simulink model "test_bu01_2018b"  (R2018b)
settings: Solver=FixedStepAuto  StartTime=0.0  StopTime=10  FixedStep=0.02  RelTol=1e-3
model workspace (MAT data in the model file):
  Ixx = 0.8
  Iyy = 2.075
  Izz = 1.25
  K = 0.75
  Mass = 11.5
  b = 0
libraries: simulink x10, aerolibutil x6, vrlib x4, sharedtransform x4, sharedutil x3, shared6dof x1
(part 1 of 4)
settings Model: Creator=Administrator  LastModifiedBy=39926
settings DataIOCC: ReturnWorkspaceOutputs=on

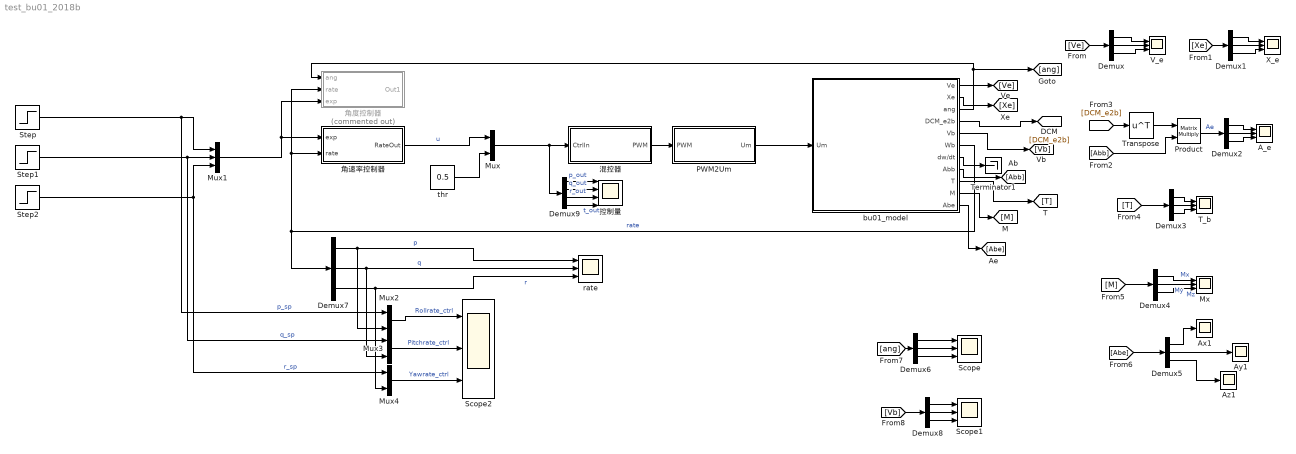
== system test_bu01_2018b ==
  A_e : Scope  NumInputPorts=3
  Ax1 : Scope
  Ay1 : Scope
  Az1 : Scope
  Demux{,1..8} (9 alike) : Demux  Outputs=3
  Demux9 : Demux
  Mux{,2..4} (4 alike) : Mux  Inputs=2
  Mux1 : Mux  Inputs=3
  Mx : Scope  NumInputPorts=3
  PWM2Um : Subsystem
  Product : Product  Multiplication=Matrix(*)
  Scope : Scope  NumInputPorts=3
  Scope1 : Scope  NumInputPorts=3
  Scope2 : Scope  NumInputPorts=3
  Step : Step  SampleTime=0
  Step1 : Step  SampleTime=0
  Step2 : Step  SampleTime=0
  T_b : Scope  NumInputPorts=3
  Terminator1 : Terminator
  Transpose : Math  Operator=transpose  SaturateOnIntegerOverflow=on
  V_e : Scope  NumInputPorts=3
  X_e : Scope  NumInputPorts=3
  bu01_model : Subsystem  mask{Density=1.185}
      mask prompts: Density "空气密度D"
  rate : Scope  NumInputPorts=3
  thr : Constant  Value=0.5
  控制量 : Scope  NumInputPorts=4
  混控器 : Subsystem
  角度控制器 : Subsystem  Commented=on
  角速率控制器 : Subsystem
  wires:
  bu01_model/8(Abb) -> [Abb]
  bu01_model/7(dw/dt) -> Terminator1/1
  bu01_model/4(DCM_e2b) -> [DCM_e2b]
  bu01_model/5(Vb) -> [Vb]
  Mux/1 -> Demux9/1, 混控器/1(CtrlIn)
  bu01_model/3(ang) -> [ang], 角度控制器/1(ang)
  bu01_model/6(Wb) -> Demux7/1, 角速率控制器/2(rate), 角度控制器/2(rate)  "rate"
  Mux1/1 -> 角度控制器/3(exp), 角速率控制器/1(exp)
  thr/1 -> Mux/2
  bu01_model/2(Xe) -> [Xe]
  Demux/1 -> V_e/1
  bu01_model/1(Ve) -> [Ve]
  [Ve] -> Demux/1
  [Xe] -> Demux1/1
  Demux1/1 -> X_e/1
  Demux1/2 -> X_e/2
  Demux1/3 -> X_e/3
  [DCM_e2b] -> Transpose/1
  Transpose/1 -> Product/1
  [Abb] -> Product/2
  Product/1 -> Demux2/1  "Ae"
  Demux2/1 -> A_e/1
  Demux2/2 -> A_e/2
  bu01_model/9(T) -> [T]
  bu01_model/10(M) -> [M]
  Demux3/3 -> T_b/3
  Demux3/2 -> T_b/2
  Demux3/1 -> T_b/1
  [T] -> Demux3/1
  [M] -> Demux4/1
  Demux4/1 -> Mx/1  "Mx"
  Demux4/2 -> Mx/2  "My"
  Demux4/3 -> Mx/3  "Mz"
  Demux2/3 -> A_e/3
  bu01_model/11(Abe) -> [Abe]
  Demux5/3 -> Az1/1
  Demux5/2 -> Ay1/1
  Demux5/1 -> Ax1/1
  [Abe] -> Demux5/1
  Step/1 -> Mux2/1, Mux1/1  "p_sp"
  Step1/1 -> Mux3/1, Mux1/2  "q_sp"
  Step2/1 -> Mux4/1, Mux1/3  "r_sp"
  Demux/2 -> V_e/2
  Demux/3 -> V_e/3
  [ang] -> Demux6/1
  Demux6/1 -> Scope/1
  Demux6/2 -> Scope/2
  Demux6/3 -> Scope/3
  PWM2Um/1(Um) -> bu01_model/1(Um)
  混控器/1(PWM) -> PWM2Um/1(PWM)
  Demux7/1 -> Mux2/2, rate/1  "p"
  Demux7/2 -> Mux3/2, rate/2  "q"
  Demux7/3 -> Mux4/2, rate/3  "r"
  [Vb] -> Demux8/1
  Demux8/1 -> Scope1/1
  Demux8/2 -> Scope1/2
  Demux8/3 -> Scope1/3
  Mux2/1 -> Scope2/1  "Rollrate_ctrl"
  Mux3/1 -> Scope2/2  "Pitchrate_ctrl"
  Mux4/1 -> Scope2/3  "Yawrate_ctrl"
  Demux9/1 -> 控制量/1  "p_out"
  Demux9/2 -> 控制量/2  "q_out"
  Demux9/3 -> 控制量/3  "r_out"
  Demux9/4 -> 控制量/4  "t_out"
  角速率控制器/1(RateOut) -> Mux/1  "u"

== system test_bu01_2018b/PWM2Um ==
  PWM : Inport
  Add : Sum  Inputs=+-
  Add1 : Sum  Inputs=+-
  Constant : Constant  Value=36.092
  Constant1 : Constant  Value=36.491
  Demux : Demux  Outputs=2
  Demux1 : Demux  Outputs=8
  Gain : Gain  Gain=0.0333
  Gain1 : Gain  Gain=0.0355
  Mux : Mux  Inputs=2
  Saturation : Saturate  UpperLimit=1900  LowerLimit=1200
  Scope : Scope  NumInputPorts=8
  Um : Outport
  wires:
  Demux/1 -> Gain/1
  Gain/1 -> Add/1
  Constant/1 -> Add/2
  Demux/2 -> Gain1/1
  Saturation/1 -> Demux/1
  PWM/1 -> Saturation/1
  Gain1/1 -> Add1/1
  Constant1/1 -> Add1/2
  Add1/1 -> Mux/2
  Add/1 -> Mux/1
  Mux/1 -> Demux1/1, Um/1
  Demux1/1 -> Scope/1
  Demux1/2 -> Scope/2
  Demux1/3 -> Scope/3
  Demux1/4 -> Scope/4
  Demux1/5 -> Scope/5
  Demux1/6 -> Scope/6
  Demux1/7 -> Scope/7
  Demux1/8 -> Scope/8

== system test_bu01_2018b/bu01_model ==
  Um : Inport
  6DOF (Quaternion) : shared6dof/6DOF (Euler Angles)  units=Metric (MKS)  mtype=Fixed  rep=Quaternion  xme_0=[0 0 0]  Vm_0=[0 0 0]  eul_0=[0 0 0]  pm_0=[0 0 0]  mass_0=Mass  mass_e=0.5  mass_f=2.0  inertia=[Ixx 0 0; 0 Iyy 0;0 0 Izz]  inertia_e=eye(3)  inertia_f=2*eye(3)  k_quat=1.0  vre_flag=on  abi_flag=on  aMode=0  xme_statename=''  Vm_statename=''  eul_statename=''  quat_statename=''  pm_statename=''  mass_statename=''
      settings: SourceProductBaseCode=AE
  Add : Sum  Inputs=3
  Add1 : Sum
  Constant : Constant  Value=Density
  Constant1 : Constant  Value=[0 0 0]
  Constant2 : Constant  Value=[0 0 0]
  动力系统模型 : Subsystem
  空气动力模型 : ModelReference  ModelNameDialog=BU01AM.slx  SimulationMode=Normal  ModelReferenceVersion=1.55
  重力模型 : Subsystem  mask{G=9.81, m=11.5}
      mask prompts: G "重力加速度G"; m "质量m"
  Ve : Outport
  Xe : Outport  Port=2
  ang : Outport  Port=3
  DCM_e2b : Outport  Port=4
  Vb : Outport  Port=5
  Wb : Outport  Port=6
  dw/dt : Outport  Port=7
  Abb : Outport  Port=8
  T : Outport  Port=9
  M : Outport  Port=10
  Abe : Outport  Port=11
  wires:
  Add1/1 -> M/1, 6DOF (Quaternion)/2  "M"
  6DOF (Quaternion)/1 -> Ve/1
  6DOF (Quaternion)/3 -> ang/1
  6DOF (Quaternion)/2 -> Xe/1
  6DOF (Quaternion)/4 -> 重力模型/1(DCM_e2b), DCM_e2b/1
  Add/1 -> T/1, 6DOF (Quaternion)/1  "T"
  6DOF (Quaternion)/7 -> dw/dt/1
  6DOF (Quaternion)/8 -> Abb/1
  6DOF (Quaternion)/5 -> Vb/1
  6DOF (Quaternion)/6 -> Wb/1, 空气动力模型/2
  Um/1 -> 动力系统模型/1("Um ")
  6DOF (Quaternion)/9 -> Abe/1
  Constant/1 -> 空气动力模型/4
  重力模型/1(Fb_mg) -> Add/1
  动力系统模型/1(Fb) -> Add/2
  空气动力模型/1 -> Add/3
  空气动力模型/2 -> Add1/2
  动力系统模型/2(Mb) -> Add1/1
  Constant1/1 -> 空气动力模型/3, 动力系统模型/3(Wb)
  Constant2/1 -> 空气动力模型/1, 动力系统模型/2(Vb)

== system test_bu01_2018b/混控器 ==
  note: 机体构型描述：
      |           ^
      |           ||
      | 1P   -  ||  -   4N
      | 2N   -  ||  -   3P
      |            ||
      |            ||
      | -------------------
      | 5N  6N   7N 8N
  CtrlIn : Inport
  Add : Sum
  Bias{1..4} (4 alike) : Bias  Bias=[0 b 0 b]
  Constant : Constant  Value=1200
  Demux : Demux  Outputs=8
  Gain : Gain  Gain="[1 1  -1 1]"
  Gain1 : Gain  Gain="[1 0  1 1]"
  Gain{7,9..11} (4 alike) : Gain  Gain=K
  Gain12 : Gain  Gain=700
  Gain2 : Gain  Gain=[-1 0 -1 1]
  Gain3 : Gain  Gain=[-1 1 1 1]
  Gain{4..6,8} (4 alike) : Gain  Gain=[0 -1 0 1]
  Mux : Mux  Inputs=8
  Saturation : Saturate  UpperLimit=1  LowerLimit=0
  Scope : Scope
  Scope1 : Scope  NumInputPorts=8
  Sum of Elements{,1..7} (8 alike) : Sum  Inputs=+
  PWM : Outport
  wires:
  Sum of Elements/1 -> Mux/1
  Gain/1 -> Sum of Elements/1
  Gain2/1 -> Sum of Elements2/1
  Gain3/1 -> Sum of Elements3/1
  Gain1/1 -> Sum of Elements1/1
  Bias3/1 -> Sum of Elements7/1
  Saturation/1 -> Gain12/1, Demux/1
  Sum of Elements1/1 -> Mux/2
  Sum of Elements2/1 -> Mux/3
  Sum of Elements3/1 -> Mux/4
  Sum of Elements4/1 -> Mux/5
  Sum of Elements5/1 -> Mux/6
  Sum of Elements6/1 -> Mux/7
  Sum of Elements7/1 -> Mux/8
  CtrlIn/1 -> Scope/1, Gain3/1, Gain4/1, Gain5/1, Gain8/1, Gain6/1, Gain1/1, Gain/1, Gain2/1
  Demux/1 -> Scope1/1  "m1"
  Demux/2 -> Scope1/2  "m2"
  Demux/3 -> Scope1/3  "m3"
  Demux/4 -> Scope1/4  "m4"
  Demux/5 -> Scope1/5  "m5"
  Demux/6 -> Scope1/6  "m6"
  Demux/7 -> Scope1/7  "m7"
  Demux/8 -> Scope1/8  "m8"
  Gain7/1 -> Bias3/1
  Gain8/1 -> Gain7/1
  Bias1/1 -> Sum of Elements6/1
  Gain6/1 -> Gain9/1
  Gain9/1 -> Bias1/1
  Bias2/1 -> Sum of Elements5/1
  Gain5/1 -> Gain10/1
  Gain10/1 -> Bias2/1
  Bias4/1 -> Sum of Elements4/1
  Gain4/1 -> Gain11/1
  Gain11/1 -> Bias4/1
  Gain12/1 -> Add/1
  Constant/1 -> Add/2
  Add/1 -> PWM/1
  Mux/1 -> Saturation/1

== system test_bu01_2018b/角度控制器 ==
  ang : Inport
  rate : Inport  Port=2
  exp : Inport  Port=3
  Demux : Demux  Outputs=3
  Demux1 : Demux  Outputs=3
  Demux2 : Demux  Outputs=3
  Mux : Mux  Inputs=3
  Mux1 : Mux  Inputs=2
  Mux2 : Mux  Inputs=2
  Mux3 : Mux  Inputs=2
  Mux4 : Mux  Inputs=3
  PID Controller : simulink/Continuous/PID Controller  Controller=PID  Form=Parallel  TimeDomain=Continuous-time  SampleTime=-1  IntegratorMethod=Forward Euler  FilterMethod=Forward Euler  ControllerParametersSource=internal  P=0.1  I=0.1  D=0  UseFilter=on  N=100  TunerSelectOption=Transfer Function Based (PID Tuner App)  InitialConditionSource=internal  InitialConditionForIntegrator=0  InitialConditionForFilter=0  DifferentiatorICPrevScaledInput=0  ExternalReset=none  TrackingMode=off  Kt=1  LimitOutput=off  UpperSaturationLimit=inf  LowerSaturationLimit=-inf  LinearizeAsGain=on  AntiWindupMode=none  Kb=1  POutMin=[]  POutMax=[]  IOutMin=[]  IOutMax=[]  DOutMin=[]  DOutMax=[]  NOutMin=[]  NOutMax=[]  SumOutMin=[]  SumOutMax=[]  SaturationOutMin=[]  SaturationOutMax=[]  PParamMin=[]  PParamMax=[]  IParamMin=[]  IParamMax=[]  DParamMin=[]  DParamMax=[]  NParamMin=[]  NParamMax=[]  KbParamMin=[]  KbParamMax=[]  KtParamMin=[]  KtParamMax=[]  KbOutMin=[]  KbOutMax=[]  KtOutMin=[]  KtOutMax=[]  IntegratorOutMin=[]  IntegratorOutMax=[]  FilterOutMin=[]  FilterOutMax=[]  SumI1OutMin=[]  SumI1OutMax=[]  SumI2OutMin=[]  SumI2OutMax=[]  SumI3OutMin=[]  SumI3OutMax=[]  SumI4OutMin=[]  SumI4OutMax=[]  SumDOutMin=[]  SumDOutMax=[]  DifferentiatorOutMin=[]  DifferentiatorOutMax=[]  FilterDiffOutCoefMin=[]  FilterDiffOutCoefMax=[]  ReciprocalOutMin=[]  ReciprocalOutMax=[]  SumDenOutMin=[]  SumDenOutMax=[]  SumNumOutMin=[]  SumNumOutMax=[]  DivideOutMin=[]  DivideOutMax=[]  IntegratorContinuousStateAttributes=''  IntegratorStateMustResolveToSignalObject=off  IntegratorRTWStateStorageClass=Auto  FilterContinuousStateAttributes=''  FilterStateMustResolveToSignalObject=off  FilterRTWStateStorageClass=Auto  ParallelPVariant=InternalParameters  IdealPVariant=Disabled  IVariant=InternalParameters  DVariant=InternalParameters  IntegratorVariant=Continuous  SatVariant=Disabled  AWVariant=Passthrough  PCopyVariant=Disabled  TRVariant=Disabled  FdbkBlocksVariant=Forward  IdealPFdbkVariant=Disabled  SatFdbkVariant=Disabled  DerivativeFilterVariant=ContFilter  NVariant=InternalParameters  NCopyVariant=Disabled  FilterICVariant=InternalICsFilter  IntegratorICVariant=InternalICs  ExternalResetVariant=Disabled  TRSumVariant=Passthrough  SumFdbkVariant=Disabled  SumVariant=Sum_PID
  PID Controller1 : simulink/Continuous/PID Controller  Controller=PID  Form=Parallel  TimeDomain=Continuous-time  SampleTime=-1  IntegratorMethod=Forward Euler  FilterMethod=Forward Euler  ControllerParametersSource=internal  P=0.15  I=0.1  D=0  UseFilter=on  N=100  TunerSelectOption=Transfer Function Based (PID Tuner App)  InitialConditionSource=internal  InitialConditionForIntegrator=0  InitialConditionForFilter=0  DifferentiatorICPrevScaledInput=0  ExternalReset=none  TrackingMode=off  Kt=1  LimitOutput=off  UpperSaturationLimit=inf  LowerSaturationLimit=-inf  LinearizeAsGain=on  AntiWindupMode=none  Kb=1  POutMin=[]  POutMax=[]  IOutMin=[]  IOutMax=[]  DOutMin=[]  DOutMax=[]  NOutMin=[]  NOutMax=[]  SumOutMin=[]  SumOutMax=[]  SaturationOutMin=[]  SaturationOutMax=[]  PParamMin=[]  PParamMax=[]  IParamMin=[]  IParamMax=[]  DParamMin=[]  DParamMax=[]  NParamMin=[]  NParamMax=[]  KbParamMin=[]  KbParamMax=[]  KtParamMin=[]  KtParamMax=[]  KbOutMin=[]  KbOutMax=[]  KtOutMin=[]  KtOutMax=[]  IntegratorOutMin=[]  IntegratorOutMax=[]  FilterOutMin=[]  FilterOutMax=[]  SumI1OutMin=[]  SumI1OutMax=[]  SumI2OutMin=[]  SumI2OutMax=[]  SumI3OutMin=[]  SumI3OutMax=[]  SumI4OutMin=[]  SumI4OutMax=[]  SumDOutMin=[]  SumDOutMax=[]  DifferentiatorOutMin=[]  DifferentiatorOutMax=[]  FilterDiffOutCoefMin=[]  FilterDiffOutCoefMax=[]  ReciprocalOutMin=[]  ReciprocalOutMax=[]  SumDenOutMin=[]  SumDenOutMax=[]  SumNumOutMin=[]  SumNumOutMax=[]  DivideOutMin=[]  DivideOutMax=[]  IntegratorContinuousStateAttributes=''  IntegratorStateMustResolveToSignalObject=off  IntegratorRTWStateStorageClass=Auto  FilterContinuousStateAttributes=''  FilterStateMustResolveToSignalObject=off  FilterRTWStateStorageClass=Auto  ParallelPVariant=InternalParameters  IdealPVariant=Disabled  IVariant=InternalParameters  DVariant=InternalParameters  IntegratorVariant=Continuous  SatVariant=Disabled  AWVariant=Passthrough  PCopyVariant=Disabled  TRVariant=Disabled  FdbkBlocksVariant=Forward  IdealPFdbkVariant=Disabled  SatFdbkVariant=Disabled  DerivativeFilterVariant=ContFilter  NVariant=InternalParameters  NCopyVariant=Disabled  FilterICVariant=InternalICsFilter  IntegratorICVariant=InternalICs  ExternalResetVariant=Disabled  TRSumVariant=Passthrough  SumFdbkVariant=Disabled  SumVariant=Sum_PID
  PID Controller2 : simulink/Continuous/PID Controller  Controller=PID  Form=Parallel  TimeDomain=Continuous-time  SampleTime=-1  IntegratorMethod=Forward Euler  FilterMethod=Forward Euler  ControllerParametersSource=internal  P=0.3  I=0.1  D=0  UseFilter=on  N=100  TunerSelectOption=Transfer Function Based (PID Tuner App)  InitialConditionSource=internal  InitialConditionForIntegrator=0  InitialConditionForFilter=0  DifferentiatorICPrevScaledInput=0  ExternalReset=none  TrackingMode=off  Kt=1  LimitOutput=off  UpperSaturationLimit=inf  LowerSaturationLimit=-inf  LinearizeAsGain=on  AntiWindupMode=none  Kb=1  POutMin=[]  POutMax=[]  IOutMin=[]  IOutMax=[]  DOutMin=[]  DOutMax=[]  NOutMin=[]  NOutMax=[]  SumOutMin=[]  SumOutMax=[]  SaturationOutMin=[]  SaturationOutMax=[]  PParamMin=[]  PParamMax=[]  IParamMin=[]  IParamMax=[]  DParamMin=[]  DParamMax=[]  NParamMin=[]  NParamMax=[]  KbParamMin=[]  KbParamMax=[]  KtParamMin=[]  KtParamMax=[]  KbOutMin=[]  KbOutMax=[]  KtOutMin=[]  KtOutMax=[]  IntegratorOutMin=[]  IntegratorOutMax=[]  FilterOutMin=[]  FilterOutMax=[]  SumI1OutMin=[]  SumI1OutMax=[]  SumI2OutMin=[]  SumI2OutMax=[]  SumI3OutMin=[]  SumI3OutMax=[]  SumI4OutMin=[]  SumI4OutMax=[]  SumDOutMin=[]  SumDOutMax=[]  DifferentiatorOutMin=[]  DifferentiatorOutMax=[]  FilterDiffOutCoefMin=[]  FilterDiffOutCoefMax=[]  ReciprocalOutMin=[]  ReciprocalOutMax=[]  SumDenOutMin=[]  SumDenOutMax=[]  SumNumOutMin=[]  SumNumOutMax=[]  DivideOutMin=[]  DivideOutMax=[]  IntegratorContinuousStateAttributes=''  IntegratorStateMustResolveToSignalObject=off  IntegratorRTWStateStorageClass=Auto  FilterContinuousStateAttributes=''  FilterStateMustResolveToSignalObject=off  FilterRTWStateStorageClass=Auto  ParallelPVariant=InternalParameters  IdealPVariant=Disabled  IVariant=InternalParameters  DVariant=InternalParameters  IntegratorVariant=Continuous  SatVariant=Disabled  AWVariant=Passthrough  PCopyVariant=Disabled  TRVariant=Disabled  FdbkBlocksVariant=Forward  IdealPFdbkVariant=Disabled  SatFdbkVariant=Disabled  DerivativeFilterVariant=ContFilter  NVariant=InternalParameters  NCopyVariant=Disabled  FilterICVariant=InternalICsFilter  IntegratorICVariant=InternalICs  ExternalResetVariant=Disabled  TRSumVariant=Passthrough  SumFdbkVariant=Disabled  SumVariant=Sum_PID
  Product : Product
  Saturation : Saturate  UpperLimit=1  LowerLimit=-1
  Scope : Scope  NumInputPorts=3
  Scope1 : Scope
  Scope2 : Scope
  Subsystem : Subsystem
  Sum : Sum  Inputs=|+-
  pitch gain : Constant
  roll gain : Constant
  yaw gain : Constant
  求取航向衰减后的期望四元数 : Subsystem
  求取角度误差 : Subsystem
  Out1 : Outport
  wires:
  ang/1 -> Demux/1, 求取航向衰减后的期望四元数/1(ang)
  exp/1 -> Demux1/1, 求取航向衰减后的期望四元数/2(exp)
  roll gain/1 -> Mux/1, Subsystem/1(roll_gain)
  pitch gain/1 -> Subsystem/2("pitch_gain "), Mux/2
  yaw gain/1 -> Subsystem/3(yaw_gain), Mux/3
  Subsystem/1(yaw_w) -> 求取航向衰减后的期望四元数/3("yaw_w ")
  求取航向衰减后的期望四元数/1(q) -> 求取角度误差/1(q)
  求取航向衰减后的期望四元数/2(qd) -> 求取角度误差/2(qd)
  求取角度误差/1(rpy_err) -> Product/1
  Mux/1 -> Product/2
  Product/1 -> Sum/1  "rate_sp"
  rate/1 -> Sum/2
  Sum/1 -> Scope1/1, Demux2/1
  Mux4/1 -> Scope2/1, Saturation/1
  Saturation/1 -> Out1/1
  Demux/1 -> Mux1/1  "roll"
  Demux1/1 -> Mux1/2  "roll_sp"
  Demux/2 -> Mux2/1  "pitch"
  Demux1/2 -> Mux2/2  "pitch_sp"
  Demux/3 -> Mux3/1  "yaw"
  Demux1/3 -> Mux3/2  "yaw_sp"
  Mux1/1 -> Scope/1
  Mux2/1 -> Scope/2
  Mux3/1 -> Scope/3
  Demux2/1 -> PID Controller/1
  Demux2/2 -> PID Controller1/1
  Demux2/3 -> PID Controller2/1
  PID Controller/1 -> Mux4/1
  PID Controller1/1 -> Mux4/2
  PID Controller2/1 -> Mux4/3

== system test_bu01_2018b/角速率控制器 ==
  exp : Inport
  rate : Inport  Port=2
  " roll-off" : TransferFcn  Numerator=[40]  Denominator=[1 40]
  " roll-off1" : TransferFcn  Numerator=[40]  Denominator=[1 40]
  " roll-off2" : TransferFcn  Numerator=[40]  Denominator=[1 40]
  Demux : Demux  Outputs=3
  Mux : Mux  Inputs=3
  PID Controller : simulink/Continuous/PID Controller  Controller=PI  Form=Parallel  TimeDomain=Continuous-time  SampleTime=-1  IntegratorMethod=Forward Euler  FilterMethod=Forward Euler  ControllerParametersSource=internal  P=0.1  I=0.01  D=0.001  UseFilter=on  N=100  TunerSelectOption=Transfer Function Based (PID Tuner App)  InitialConditionSource=internal  InitialConditionForIntegrator=0  InitialConditionForFilter=0  DifferentiatorICPrevScaledInput=0  ExternalReset=none  TrackingMode=off  Kt=1  LimitOutput=off  UpperSaturationLimit=1  LowerSaturationLimit=-1  LinearizeAsGain=on  AntiWindupMode=none  Kb=1  POutMin=[]  POutMax=[]  IOutMin=[]  IOutMax=[]  DOutMin=[]  DOutMax=[]  NOutMin=[]  NOutMax=[]  SumOutMin=[]  SumOutMax=[]  SaturationOutMin=[]  SaturationOutMax=[]  PParamMin=[]  PParamMax=[]  IParamMin=[]  IParamMax=[]  DParamMin=[]  DParamMax=[]  NParamMin=[]  NParamMax=[]  KbParamMin=[]  KbParamMax=[]  KtParamMin=[]  KtParamMax=[]  KbOutMin=[]  KbOutMax=[]  KtOutMin=[]  KtOutMax=[]  IntegratorOutMin=[]  IntegratorOutMax=[]  FilterOutMin=[]  FilterOutMax=[]  SumI1OutMin=[]  SumI1OutMax=[]  SumI2OutMin=[]  SumI2OutMax=[]  SumI3OutMin=[]  SumI3OutMax=[]  SumI4OutMin=[]  SumI4OutMax=[]  SumDOutMin=[]  SumDOutMax=[]  DifferentiatorOutMin=[]  DifferentiatorOutMax=[]  FilterDiffOutCoefMin=[]  FilterDiffOutCoefMax=[]  ReciprocalOutMin=[]  ReciprocalOutMax=[]  SumDenOutMin=[]  SumDenOutMax=[]  SumNumOutMin=[]  SumNumOutMax=[]  DivideOutMin=[]  DivideOutMax=[]  IntegratorContinuousStateAttributes=''  IntegratorStateMustResolveToSignalObject=off  IntegratorRTWStateStorageClass=Auto  FilterContinuousStateAttributes=''  FilterStateMustResolveToSignalObject=off  FilterRTWStateStorageClass=Auto  ParallelPVariant=InternalParameters  IdealPVariant=Disabled  IVariant=InternalParameters  DVariant=Disabled  IntegratorVariant=Continuous  SatVariant=Disabled  AWVariant=Passthrough  PCopyVariant=Disabled  TRVariant=Disabled  FdbkBlocksVariant=Forward  IdealPFdbkVariant=Disabled  SatFdbkVariant=Disabled  DerivativeFilterVariant=Disabled  NVariant=Disabled  NCopyVariant=Disabled_SignalSpec  FilterICVariant=Disabled  IntegratorICVariant=InternalICs  ExternalResetVariant=Disabled  TRSumVariant=Passthrough  SumFdbkVariant=Disabled  SumVariant=Sum_PI
  PID Controller1 : simulink/Continuous/PID Controller  Controller=PI  Form=Parallel  TimeDomain=Continuous-time  SampleTime=-1  IntegratorMethod=Forward Euler  FilterMethod=Forward Euler  ControllerParametersSource=internal  P=0.1  I=0.01  D=0  UseFilter=on  N=100  TunerSelectOption=Transfer Function Based (PID Tuner App)  InitialConditionSource=internal  InitialConditionForIntegrator=0  InitialConditionForFilter=0  DifferentiatorICPrevScaledInput=0  ExternalReset=none  TrackingMode=off  Kt=1  LimitOutput=off  UpperSaturationLimit=1  LowerSaturationLimit=-1  LinearizeAsGain=on  AntiWindupMode=none  Kb=1  POutMin=[]  POutMax=[]  IOutMin=[]  IOutMax=[]  DOutMin=[]  DOutMax=[]  NOutMin=[]  NOutMax=[]  SumOutMin=[]  SumOutMax=[]  SaturationOutMin=[]  SaturationOutMax=[]  PParamMin=[]  PParamMax=[]  IParamMin=[]  IParamMax=[]  DParamMin=[]  DParamMax=[]  NParamMin=[]  NParamMax=[]  KbParamMin=[]  KbParamMax=[]  KtParamMin=[]  KtParamMax=[]  KbOutMin=[]  KbOutMax=[]  KtOutMin=[]  KtOutMax=[]  IntegratorOutMin=[]  IntegratorOutMax=[]  FilterOutMin=[]  FilterOutMax=[]  SumI1OutMin=[]  SumI1OutMax=[]  SumI2OutMin=[]  SumI2OutMax=[]  SumI3OutMin=[]  SumI3OutMax=[]  SumI4OutMin=[]  SumI4OutMax=[]  SumDOutMin=[]  SumDOutMax=[]  DifferentiatorOutMin=[]  DifferentiatorOutMax=[]  FilterDiffOutCoefMin=[]  FilterDiffOutCoefMax=[]  ReciprocalOutMin=[]  ReciprocalOutMax=[]  SumDenOutMin=[]  SumDenOutMax=[]  SumNumOutMin=[]  SumNumOutMax=[]  DivideOutMin=[]  DivideOutMax=[]  IntegratorContinuousStateAttributes=''  IntegratorStateMustResolveToSignalObject=off  IntegratorRTWStateStorageClass=Auto  FilterContinuousStateAttributes=''  FilterStateMustResolveToSignalObject=off  FilterRTWStateStorageClass=Auto  ParallelPVariant=InternalParameters  IdealPVariant=Disabled  IVariant=InternalParameters  DVariant=Disabled  IntegratorVariant=Continuous  SatVariant=Disabled  AWVariant=Passthrough  PCopyVariant=Disabled  TRVariant=Disabled  FdbkBlocksVariant=Forward  IdealPFdbkVariant=Disabled  SatFdbkVariant=Disabled  DerivativeFilterVariant=Disabled  NVariant=Disabled  NCopyVariant=Disabled_SignalSpec  FilterICVariant=Disabled  IntegratorICVariant=InternalICs  ExternalResetVariant=Disabled  TRSumVariant=Passthrough  SumFdbkVariant=Disabled  SumVariant=Sum_PI
  PID Controller2 : simulink/Continuous/PID Controller  Controller=PI  Form=Parallel  TimeDomain=Continuous-time  SampleTime=-1  IntegratorMethod=Forward Euler  FilterMethod=Forward Euler  ControllerParametersSource=internal  P=0.1  I=0.01  D=0  UseFilter=on  N=100  TunerSelectOption=Transfer Function Based (PID Tuner App)  InitialConditionSource=internal  InitialConditionForIntegrator=0  InitialConditionForFilter=0  DifferentiatorICPrevScaledInput=0  ExternalReset=none  TrackingMode=off  Kt=1  LimitOutput=off  UpperSaturationLimit=1  LowerSaturationLimit=-1  LinearizeAsGain=on  AntiWindupMode=none  Kb=1  POutMin=[]  POutMax=[]  IOutMin=[]  IOutMax=[]  DOutMin=[]  DOutMax=[]  NOutMin=[]  NOutMax=[]  SumOutMin=[]  SumOutMax=[]  SaturationOutMin=[]  SaturationOutMax=[]  PParamMin=[]  PParamMax=[]  IParamMin=[]  IParamMax=[]  DParamMin=[]  DParamMax=[]  NParamMin=[]  NParamMax=[]  KbParamMin=[]  KbParamMax=[]  KtParamMin=[]  KtParamMax=[]  KbOutMin=[]  KbOutMax=[]  KtOutMin=[]  KtOutMax=[]  IntegratorOutMin=[]  IntegratorOutMax=[]  FilterOutMin=[]  FilterOutMax=[]  SumI1OutMin=[]  SumI1OutMax=[]  SumI2OutMin=[]  SumI2OutMax=[]  SumI3OutMin=[]  SumI3OutMax=[]  SumI4OutMin=[]  SumI4OutMax=[]  SumDOutMin=[]  SumDOutMax=[]  DifferentiatorOutMin=[]  DifferentiatorOutMax=[]  FilterDiffOutCoefMin=[]  FilterDiffOutCoefMax=[]  ReciprocalOutMin=[]  ReciprocalOutMax=[]  SumDenOutMin=[]  SumDenOutMax=[]  SumNumOutMin=[]  SumNumOutMax=[]  DivideOutMin=[]  DivideOutMax=[]  IntegratorContinuousStateAttributes=''  IntegratorStateMustResolveToSignalObject=off  IntegratorRTWStateStorageClass=Auto  FilterContinuousStateAttributes=''  FilterStateMustResolveToSignalObject=off  FilterRTWStateStorageClass=Auto  ParallelPVariant=InternalParameters  IdealPVariant=Disabled  IVariant=InternalParameters  DVariant=Disabled  IntegratorVariant=Continuous  SatVariant=Disabled  AWVariant=Passthrough  PCopyVariant=Disabled  TRVariant=Disabled  FdbkBlocksVariant=Forward  IdealPFdbkVariant=Disabled  SatFdbkVariant=Disabled  DerivativeFilterVariant=Disabled  NVariant=Disabled  NCopyVariant=Disabled_SignalSpec  FilterICVariant=Disabled  IntegratorICVariant=InternalICs  ExternalResetVariant=Disabled  TRSumVariant=Passthrough  SumFdbkVariant=Disabled  SumVariant=Sum_PI
  Sum : Sum  Inputs=|+-
  RateOut : Outport
  wires:
  Mux/1 -> RateOut/1
  exp/1 -> Sum/1
  rate/1 -> Sum/2
  Sum/1 -> Demux/1
  Demux/1 -> PID Controller/1
  Demux/2 -> PID Controller1/1
  Demux/3 -> PID Controller2/1
  PID Controller/1 -> " roll-off"/1
  " roll-off"/1 -> Mux/1
  " roll-off1"/1 -> Mux/2
  PID Controller1/1 -> " roll-off1"/1
  PID Controller2/1 -> " roll-off2"/1
  " roll-off2"/1 -> Mux/3

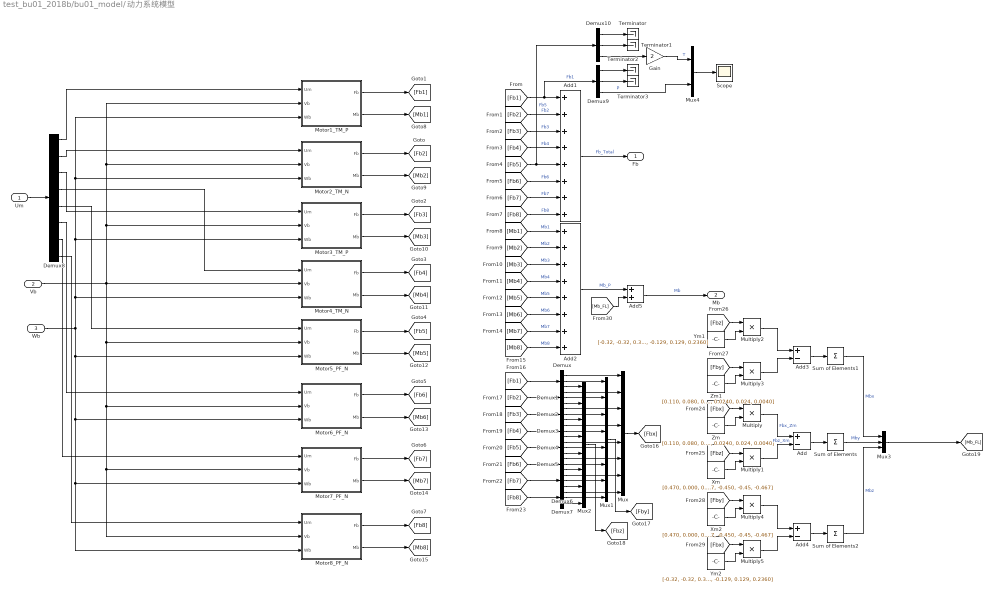
== system test_bu01_2018b/bu01_model/动力系统模型 ==
  "Um " : Inport
  Vb : Inport  Port=2
  Wb : Inport  Port=3
  Add : Sum  Inputs=+-
  Add1 : Sum  Inputs=8
  Add2 : Sum  Inputs=8
  Add3 : Sum  Inputs=+-
  Add4 : Sum  Inputs=+-
  Add5 : Sum
  Demux{,1..7,9..10} (10 alike) : Demux  Outputs=3
  Demux8 : Demux  Outputs=8
  Gain : Gain  Gain=2
  Motor1_TM_P : Subsystem
  Motor2_TM_N : Subsystem
  Motor3_TM_P : Subsystem
  Motor4_TM_N : Subsystem
  Motor5_PF_N : Subsystem
  Motor6_PF_N : Subsystem
  Motor7_PF_N : Subsystem
  Motor8_PF_N : Subsystem
  Multiply{,1..5} (6 alike) : Product
  Mux : Mux  Inputs=8
  Mux1 : Mux  Inputs=8
  Mux2 : Mux  Inputs=8
  Mux3 : Mux  Inputs=3
  Mux4 : Mux  Inputs=2
  Scope : Scope
  Sum of Elements : Sum  Inputs=+
  Sum of Elements1 : Sum  Inputs=+
  Sum of Elements2 : Sum  Inputs=+
  Terminator{,1..3} (4 alike) : Terminator
  Xm : Constant  Value=[0.470, 0.000, 0.00, 0.47, -0.467, -0.450, -0.45, -0.467]
  Xm2 : Constant  Value=[0.470, 0.000, 0.00, 0.47, -0.467, -0.450, -0.45, -0.467]
  Ym1 : Constant  Value=[-0.32, -0.32, 0.32, 0.32, -0.236, -0.129, 0.129, 0.2360]
  Ym2 : Constant  Value=[-0.32, -0.32, 0.32, 0.32, -0.236, -0.129, 0.129, 0.2360]
  Zm : Constant  Value=[0.110, 0.080, 0.08, 0.11, 0.0040, 0.0240, 0.024, 0.0040]
  Zm1 : Constant  Value=[0.110, 0.080, 0.08, 0.11, 0.0040, 0.0240, 0.024, 0.0040]
  Fb : Outport
  Mb : Outport  Port=2
  wires:
  Mux4/1 -> Scope/1
  Gain/1 -> Mux4/1  "T"
  Demux10/3 -> Gain/1
  Demux9/3 -> Mux4/2  "P"
  Demux9/2 -> Terminator3/1
  Demux9/1 -> Terminator2/1
  Demux10/2 -> Terminator1/1
  Demux10/1 -> Terminator/1
  Vb/1 -> Motor4_TM_N/2(Vb), Motor3_TM_P/2(Vb), Motor1_TM_P/2(Vb), Motor2_TM_N/2(Vb), Motor5_PF_N/2(Vb), Motor6_PF_N/2(Vb), Motor8_PF_N/2(Vb), Motor7_PF_N/2(Vb)
  Wb/1 -> Motor5_PF_N/3(Wb), Motor6_PF_N/3(Wb), Motor8_PF_N/3(Wb), Motor7_PF_N/3(Wb), Motor4_TM_N/3(Wb), Motor3_TM_P/3(Wb), Motor1_TM_P/3(Wb), Motor2_TM_N/3(Wb)
  Motor1_TM_P/1(Fb) -> [Fb1]
  Motor2_TM_N/1(Fb) -> [Fb2]
  Motor3_TM_P/1(Fb) -> [Fb3]
  Motor4_TM_N/1(Fb) -> [Fb4]
  Motor5_PF_N/1(Fb) -> [Fb5]
  Motor6_PF_N/1(Fb) -> [Fb6]
  Motor7_PF_N/1(Fb) -> [Fb7]
  Motor8_PF_N/1(Fb) -> [Fb8]
  Motor1_TM_P/2(Mb) -> [Mb1]
  Motor3_TM_P/2(Mb) -> [Mb3]
  Motor4_TM_N/2(Mb) -> [Mb4]
  Motor5_PF_N/2(Mb) -> [Mb5]
  Motor6_PF_N/2(Mb) -> [Mb6]
  Motor7_PF_N/2(Mb) -> [Mb7]
  Motor8_PF_N/2(Mb) -> [Mb8]
  [Fb8] -> Add1/8  "Fb8"
  [Fb7] -> Add1/7  "Fb7"
  [Fb6] -> Add1/6  "Fb6"
  [Fb5] -> Add1/5, Demux10/1  "Fb5"
  [Fb4] -> Add1/4  "Fb4"
  [Fb3] -> Add1/3  "Fb3"
  [Fb2] -> Add1/2  "Fb2"
  [Fb1] -> Add1/1, Demux9/1  "Fb1"
  Add1/1 -> Fb/1  "Fb_Total"
  [Mb1] -> Add2/1  "Mb1"
  [Mb4] -> Add2/4  "Mb4"
  [Mb3] -> Add2/3  "Mb3"
  [Mb2] -> Add2/2  "Mb2"
  [Mb5] -> Add2/5  "Mb5"
  [Mb6] -> Add2/6  "Mb6"
  [Mb7] -> Add2/7  "Mb7"
  [Mb8] -> Add2/8  "Mb8"
  [Fb1] -> Demux/1
  [Fb3] -> Demux2/1
  [Fb7] -> Demux6/1
  [Fb8] -> Demux7/1
  [Fb2] -> Demux1/1
  [Fb4] -> Demux3/1
  [Fb6] -> Demux5/1
  [Fb5] -> Demux4/1
  Demux/1 -> Mux/1
  Demux1/1 -> Mux/2
  Demux2/1 -> Mux/3
  Demux3/1 -> Mux/4
  Demux4/1 -> Mux/5
  Demux5/1 -> Mux/6
  Demux6/1 -> Mux/7
  Demux7/1 -> Mux/8
  Demux/2 -> Mux1/1
  Demux1/2 -> Mux1/2
  Demux2/2 -> Mux1/3
  Demux3/2 -> Mux1/4
  Demux4/2 -> Mux1/5
  Demux5/2 -> Mux1/6
  Demux6/2 -> Mux1/7
  Demux7/2 -> Mux1/8
  Demux/3 -> Mux2/1
  Demux1/3 -> Mux2/2
  Demux2/3 -> Mux2/3
  Demux3/3 -> Mux2/4
  Demux4/3 -> Mux2/5
  Demux5/3 -> Mux2/6
  Demux6/3 -> Mux2/7
  Demux7/3 -> Mux2/8
  Mux/1 -> [Fbx]
  Mux1/1 -> [Fby]
  Mux2/1 -> [Fbz]
  [Fbx] -> Multiply/1
  Zm/1 -> Multiply/2
  Multiply/1 -> Add/1  "Fbx_Zm"
  [Fbz] -> Multiply1/1
  Xm/1 -> Multiply1/2
  Multiply1/1 -> Add/2  "Fbz_Xm"
  Add/1 -> Sum of Elements/1
  Sum of Elements/1 -> Mux3/2  "Mby"
  [Fbz] -> Multiply2/1
  Multiply2/1 -> Add3/1
  Zm1/1 -> Multiply3/2
  [Fby] -> Multiply3/1
  Ym1/1 -> Multiply2/2
  Sum of Elements1/1 -> Mux3/1  "Mbx"
  Add3/1 -> Sum of Elements1/1
  Multiply3/1 -> Add3/2
  [Fby] -> Multiply4/1
  Multiply4/1 -> Add4/1
  Ym2/1 -> Multiply5/2
  [Fbx] -> Multiply5/1
  Xm2/1 -> Multiply4/2
  Sum of Elements2/1 -> Mux3/3  "Mbz"
  Add4/1 -> Sum of Elements2/1
  Multiply5/1 -> Add4/2
  Mux3/1 -> [Mb_FL]
  [Mb_FL] -> Add5/2
  Add2/1 -> Add5/1  "Mb_P"
  Add5/1 -> Mb/1  "Mb"
  "Um "/1 -> Demux8/1
  Demux8/1 -> Motor1_TM_P/1(Um)
  Demux8/2 -> Motor2_TM_N/1(Um)
  Demux8/3 -> Motor3_TM_P/1(Um)
  Demux8/4 -> Motor4_TM_N/1(Um)
  Demux8/5 -> Motor5_PF_N/1(Um)
  Demux8/6 -> Motor6_PF_N/1(Um)
  Demux8/7 -> Motor7_PF_N/1(Um)
  Demux8/8 -> Motor8_PF_N/1(Um)
  Motor2_TM_N/2(Mb) -> [Mb2]

== system test_bu01_2018b/bu01_model/重力模型 ==
  DCM_e2b : Inport
  Constant : Constant  Value=[0 0 m*G]
  Multiply : Product  Multiplication=Matrix(*)
  Fb_mg : Outport
  wires:
  DCM_e2b/1 -> Multiply/1
  Constant/1 -> Multiply/2
  Multiply/1 -> Fb_mg/1

== system test_bu01_2018b/角度控制器/Subsystem ==
  note: 将比例增益当做系统时间常数，用其比例关系作为控制器衰减比例
  roll_gain : Inport
  "pitch_gain " : Inport  Port=2
  yaw_gain : Inport  Port=3
  Add : Sum
  Divide : Product  Inputs=*/
  Gain : Gain  Gain=0.5
  Saturation : Saturate  UpperLimit=1  LowerLimit=0
  yaw_w : Outport
  wires:
  roll_gain/1 -> Add/1
  Add/1 -> Gain/1
  "pitch_gain "/1 -> Add/2
  Gain/1 -> Divide/2
  yaw_gain/1 -> Divide/1
  Divide/1 -> Saturation/1
  Saturation/1 -> yaw_w/1

== system test_bu01_2018b/角度控制器/求取航向衰减后的期望四元数 ==
  ang : Inport
  exp : Inport  Port=2
  "yaw_w " : Inport  Port=3
  MATLAB Function : MATLAB Function  TreatAsAtomicUnit=on
  Quaternion Normalize : sharedutil/Quaternion Normalize  aMode=aMode
      settings: SourceProductName=Aerospace Blockset  SourceProductBaseCode=AE
  求取只要倾斜的运动的期望四元数 : Subsystem
  求取绕机体Z轴旋转的误差四元数 : Subsystem
  获取地球系下当前机体系Z轴矢量 : Subsystem
  获取地球系下期望机体系Z轴矢量 : Subsystem
  计算航向衰减后的期望四元数 : Subsystem
  q : Outport
  qd : Outport  Port=2
  wires:
  获取地球系下当前机体系Z轴矢量/2(e_z) -> MATLAB Function/1(src)
  ang/1 -> 获取地球系下当前机体系Z轴矢量/1(ang)
  exp/1 -> 获取地球系下期望机体系Z轴矢量/1(exp)
  获取地球系下当前机体系Z轴矢量/1(q) -> q/1, 求取只要倾斜的运动的期望四元数/1(q)
  获取地球系下期望机体系Z轴矢量/1(e_z_d) -> MATLAB Function/2(dst)
  获取地球系下期望机体系Z轴矢量/2("qd ") -> 求取绕机体Z轴旋转的误差四元数/2(qd), 求取只要倾斜的运动的期望四元数/3(qd)
  "yaw_w "/1 -> 计算航向衰减后的期望四元数/1(yaw_w)
  求取绕机体Z轴旋转的误差四元数/1(q_mix_sign) -> 计算航向衰减后的期望四元数/3(q_mix_sign)
  计算航向衰减后的期望四元数/1(qd) -> qd/1
  求取只要倾斜的运动的期望四元数/1(qd_red_update) -> 计算航向衰减后的期望四元数/2(q_red_update), 求取绕机体Z轴旋转的误差四元数/1(qd_red_update)
  MATLAB Function/1(q) -> Quaternion Normalize/1  "qd_red"
  Quaternion Normalize/1 -> 求取只要倾斜的运动的期望四元数/2(qd_red)

== system test_bu01_2018b/角度控制器/求取角度误差 ==
  q : Inport
  qd : Inport  Port=2
  Constant : Constant  Value=0
  Gain : Gain  Gain=-1
  Gain1 : Gain  Gain=2
  GreaterThanOrEqual : RelationalOperator  OutDataTypeStr=boolean  RndMeth=Simplest
  Quaternion Inverse : aerolibutil/Quaternion Inverse
      settings: SourceProductName=Aerospace Blockset
  Quaternion Multiplication : aerolibutil/Quaternion Multiplication
  Selector : Selector  InputPortWidth=4  IndexOptions=Index vector (dialog)  Indices=1  OutputSizes=1
  Selector1 : Selector  InputPortWidth=4  IndexOptions=Index vector (dialog)  Indices=[2 3 4]  OutputSizes=1
  Switch : Switch  Criteria=u2 > Threshold
  rpy_err : Outport
  wires:
  Quaternion Inverse/1 -> Quaternion Multiplication/1
  q/1 -> Quaternion Inverse/1
  Quaternion Multiplication/1 -> Selector1/1, Selector/1  "quat_err"
  qd/1 -> Quaternion Multiplication/2
  Selector/1 -> GreaterThanOrEqual/1
  Constant/1 -> GreaterThanOrEqual/2
  GreaterThanOrEqual/1 -> Switch/2
  Selector1/1 -> Switch/1, Gain/1
  Gain/1 -> Switch/3
  Switch/1 -> Gain1/1
  Gain1/1 -> rpy_err/1  "ang_err"

== system test_bu01_2018b/bu01_model/动力系统模型/Motor1_TM_P ==
  Um : Inport
  Vb : Inport  Port=2
  Wb : Inport  Port=3
  Constant : Constant  Value=[0 0 -1]
  Constant1 : Constant  Value=1.185
  Gain : Gain  Gain=1/60
  "TM1654P " : Subsystem
  "TMU5KV400 " : Subsystem
  Terminator : Terminator
  Fb : Outport
  Mb : Outport  Port=2
  wires:
  Constant1/1 -> "TM1654P "/4(Density)
  Wb/1 -> "TM1654P "/2(Wb)
  Vb/1 -> "TM1654P "/1(Vb)
  Constant/1 -> "TM1654P "/3(Ax)
  "TMU5KV400 "/1(Im) -> Terminator/1
  Gain/1 -> "TM1654P "/5(Ns)
  "TMU5KV400 "/2(RPM) -> Gain/1
  "TM1654P "/2(Mb) -> Mb/1  "Mb"
  "TM1654P "/1(Fb) -> Fb/1  "Fb"
  "TM1654P "/3(Tq) -> "TMU5KV400 "/2(Tq)
  "TM1654P "/4(Izz) -> "TMU5KV400 "/3(Izz)
  Um/1 -> "TMU5KV400 "/1(Um)

== system test_bu01_2018b/bu01_model/动力系统模型/Motor2_TM_N ==
  Um : Inport
  Vb : Inport  Port=2
  Wb : Inport  Port=3
  Constant2 : Constant  Value=[0 0 -1]
  Constant3 : Constant  Value=1.185
  Gain1 : Gain  Gain=1/60
  "TM1654N " : Subsystem
  "TMU5KV400 " : Subsystem
  Terminator1 : Terminator
  Fb : Outport
  Mb : Outport  Port=2
  wires:
  Constant2/1 -> "TM1654N "/3(Ax)
  "TM1654N "/4(Izz) -> "TMU5KV400 "/3(Izz)
  "TM1654N "/1(Fb) -> Fb/1  "Fb"
  "TMU5KV400 "/1(Im) -> Terminator1/1
  Constant3/1 -> "TM1654N "/4(Density)
  "TM1654N "/3(Tq) -> "TMU5KV400 "/2(Tq)
  Wb/1 -> "TM1654N "/2(Wb)
  Gain1/1 -> "TM1654N "/5(Ns)
  Um/1 -> "TMU5KV400 "/1(Um)
  "TM1654N "/2(Mb) -> Mb/1  "Mb"
  "TMU5KV400 "/2(RPM) -> Gain1/1
  Vb/1 -> "TM1654N "/1(Vb)

== system test_bu01_2018b/bu01_model/动力系统模型/Motor3_TM_P ==
  Um : Inport
  Vb : Inport  Port=2
  Wb : Inport  Port=3
  Constant : Constant  Value=[0 0 -1]
  Constant1 : Constant  Value=1.185
  Gain : Gain  Gain=1/60
  "TM1654P " : Subsystem
  "TMU5KV400 " : Subsystem
  Terminator : Terminator
  Fb : Outport
  Mb : Outport  Port=2
  wires:
  Constant1/1 -> "TM1654P "/4(Density)
  Wb/1 -> "TM1654P "/2(Wb)
  Vb/1 -> "TM1654P "/1(Vb)
  Constant/1 -> "TM1654P "/3(Ax)
  "TMU5KV400 "/1(Im) -> Terminator/1
  Gain/1 -> "TM1654P "/5(Ns)
  "TMU5KV400 "/2(RPM) -> Gain/1
  "TM1654P "/2(Mb) -> Mb/1  "Mb"
  "TM1654P "/1(Fb) -> Fb/1  "Fb"
  "TM1654P "/3(Tq) -> "TMU5KV400 "/2(Tq)
  "TM1654P "/4(Izz) -> "TMU5KV400 "/3(Izz)
  Um/1 -> "TMU5KV400 "/1(Um)

== system test_bu01_2018b/bu01_model/动力系统模型/Motor4_TM_N ==
  Um : Inport
  Vb : Inport  Port=2
  Wb : Inport  Port=3
  Constant : Constant  Value=[0 0 -1]
  Constant3 : Constant  Value=1.185
  Gain1 : Gain  Gain=1/60
  "TM1654N " : Subsystem
  "TMU5KV400 " : Subsystem
  Terminator1 : Terminator
  Fb : Outport
  Mb : Outport  Port=2
  wires:
  Constant/1 -> "TM1654N "/3(Ax)
  "TM1654N "/4(Izz) -> "TMU5KV400 "/3(Izz)
  "TM1654N "/1(Fb) -> Fb/1  "Fb"
  "TMU5KV400 "/1(Im) -> Terminator1/1
  Constant3/1 -> "TM1654N "/4(Density)
  "TM1654N "/3(Tq) -> "TMU5KV400 "/2(Tq)
  Wb/1 -> "TM1654N "/2(Wb)
  Gain1/1 -> "TM1654N "/5(Ns)
  Um/1 -> "TMU5KV400 "/1(Um)
  "TM1654N "/2(Mb) -> Mb/1  "Mb"
  "TMU5KV400 "/2(RPM) -> Gain1/1
  Vb/1 -> "TM1654N "/1(Vb)

== system test_bu01_2018b/bu01_model/动力系统模型/Motor5_PF_N ==
  Um : Inport
  Vb : Inport  Port=2
  Wb : Inport  Port=3
  Constant : Constant  Value=[0 0 -1]
  Constant1 : Constant  Value=1.185
  Gain : Gain  Gain=1/60
  PF70mmDuctFanN : Subsystem
  PFKV2300 : Subsystem
  Terminator : Terminator
  Fb : Outport
  Mb : Outport  Port=2
  wires:
  Um/1 -> PFKV2300/1(Um)
  PF70mmDuctFanN/4(Izz) -> PFKV2300/3(Izz)
  PF70mmDuctFanN/3(Tq) -> PFKV2300/2(Tq)
  PF70mmDuctFanN/1(Fb) -> Fb/1  "Fb"
  PF70mmDuctFanN/2(Mb) -> Mb/1  "Mb"
  PFKV2300/2(RPM) -> Gain/1
  PFKV2300/1(Im) -> Terminator/1
  Constant/1 -> PF70mmDuctFanN/3(Ax_ip)
  Vb/1 -> PF70mmDuctFanN/1(Vb_ip)
  Wb/1 -> PF70mmDuctFanN/2(Wb_ip)
  Gain/1 -> PF70mmDuctFanN/4(Ns_ip)
  Constant1/1 -> PF70mmDuctFanN/5(Pro)

== system test_bu01_2018b/bu01_model/动力系统模型/Motor6_PF_N ==
  Um : Inport
  Vb : Inport  Port=2
  Wb : Inport  Port=3
  Constant : Constant  Value=[0 0 -1]
  Constant1 : Constant  Value=1.185
  Gain : Gain  Gain=1/60
  PF70mmDuctFanN : Subsystem
  PFKV2300 : Subsystem
  Terminator : Terminator
  Fb : Outport
  Mb : Outport  Port=2
  wires:
  Um/1 -> PFKV2300/1(Um)
  PF70mmDuctFanN/4(Izz) -> PFKV2300/3(Izz)
  PF70mmDuctFanN/3(Tq) -> PFKV2300/2(Tq)
  PF70mmDuctFanN/1(Fb) -> Fb/1  "Fb"
  PF70mmDuctFanN/2(Mb) -> Mb/1  "Mb"
  PFKV2300/2(RPM) -> Gain/1
  PFKV2300/1(Im) -> Terminator/1
  Constant/1 -> PF70mmDuctFanN/3(Ax_ip)
  Vb/1 -> PF70mmDuctFanN/1(Vb_ip)
  Wb/1 -> PF70mmDuctFanN/2(Wb_ip)
  Gain/1 -> PF70mmDuctFanN/4(Ns_ip)
  Constant1/1 -> PF70mmDuctFanN/5(Pro)

== system test_bu01_2018b/bu01_model/动力系统模型/Motor7_PF_N ==
  Um : Inport
  Vb : Inport  Port=2
  Wb : Inport  Port=3
  Constant : Constant  Value=[0 0 -1]
  Constant1 : Constant  Value=1.185
  Gain : Gain  Gain=1/60
  PF70mmDuctFanN : Subsystem
  PFKV2300 : Subsystem
  Terminator : Terminator
  Fb : Outport
  Mb : Outport  Port=2
  wires:
  Um/1 -> PFKV2300/1(Um)
  PF70mmDuctFanN/4(Izz) -> PFKV2300/3(Izz)
  PF70mmDuctFanN/3(Tq) -> PFKV2300/2(Tq)
  PF70mmDuctFanN/1(Fb) -> Fb/1  "Fb"
  PF70mmDuctFanN/2(Mb) -> Mb/1  "Mb"
  PFKV2300/2(RPM) -> Gain/1
  PFKV2300/1(Im) -> Terminator/1
  Constant/1 -> PF70mmDuctFanN/3(Ax_ip)
  Vb/1 -> PF70mmDuctFanN/1(Vb_ip)
  Wb/1 -> PF70mmDuctFanN/2(Wb_ip)
  Gain/1 -> PF70mmDuctFanN/4(Ns_ip)
  Constant1/1 -> PF70mmDuctFanN/5(Pro)

== system test_bu01_2018b/bu01_model/动力系统模型/Motor8_PF_N ==
  Um : Inport
  Vb : Inport  Port=2
  Wb : Inport  Port=3
  Constant : Constant  Value=[0 0 -1]
  Constant1 : Constant  Value=1.185
  Gain : Gain  Gain=1/60
  PF70mmDuctFanN : Subsystem
  PFKV2300 : Subsystem
  Terminator : Terminator
  Fb : Outport
  Mb : Outport  Port=2
  wires:
  Constant1/1 -> PF70mmDuctFanN/5(Pro)
  Gain/1 -> PF70mmDuctFanN/4(Ns_ip)
  Wb/1 -> PF70mmDuctFanN/2(Wb_ip)
  Vb/1 -> PF70mmDuctFanN/1(Vb_ip)
  Constant/1 -> PF70mmDuctFanN/3(Ax_ip)
  PFKV2300/1(Im) -> Terminator/1
  PFKV2300/2(RPM) -> Gain/1
  PF70mmDuctFanN/2(Mb) -> Mb/1  "Mb"
  PF70mmDuctFanN/1(Fb) -> Fb/1  "Fb"
  PF70mmDuctFanN/3(Tq) -> PFKV2300/2(Tq)
  PF70mmDuctFanN/4(Izz) -> PFKV2300/3(Izz)
  Um/1 -> PFKV2300/1(Um)

== system test_bu01_2018b/角度控制器/求取航向衰减后的期望四元数/求取只要倾斜的运动的期望四元数 ==
  note: 没有航向旋转的情况
  q : Inport
  qd_red : Inport  Port=2
  qd : Inport  Port=3
  Constant : Constant  Value=1-1e-5
  Demux : Demux  Outputs=2
  GreaterThan : RelationalOperator  Operator=>  OutDataTypeStr=boolean  RndMeth=Simplest
  GreaterThan1 : RelationalOperator  Operator=>  OutDataTypeStr=boolean  RndMeth=Simplest
  OR : Logic  Operator=OR  IconShape=distinctive  AllPortsSameDT=off  OutDataTypeStr=boolean
  Quaternion Multiplication : aerolibutil/Quaternion Multiplication
  Selector : Selector  InputPortWidth=4  IndexOptions=Index vector (dialog)  Indices=[2 3]  OutputSizes=1
  Switch : Switch  Criteria=u2 > Threshold
  qd_red_update : Outport
  wires:
  qd/1 -> Switch/1
  Constant/1 -> GreaterThan/2, GreaterThan1/2
  GreaterThan/1 -> OR/1
  q/1 -> Quaternion Multiplication/2
  GreaterThan1/1 -> OR/2
  qd_red/1 -> Quaternion Multiplication/1, Selector/1
  OR/1 -> Switch/2
  Demux/2 -> GreaterThan1/1
  Demux/1 -> GreaterThan/1
  Selector/1 -> Demux/1
  Quaternion Multiplication/1 -> Switch/3
  Switch/1 -> qd_red_update/1  "qd_red_update"

== system test_bu01_2018b/角度控制器/求取航向衰减后的期望四元数/求取绕机体Z轴旋转的误差四元数 ==
  qd_red_update : Inport
  qd : Inport  Port=2
  Constant1 : Constant  Value=0
  Gain : Gain  Gain=-1
  GreaterThan2 : RelationalOperator  OutDataTypeStr=boolean  RndMeth=Simplest
  Quaternion Inverse : aerolibutil/Quaternion Inverse
      settings: SourceProductName=Aerospace Blockset
  Quaternion Multiplication1 : aerolibutil/Quaternion Multiplication
  Selector1 : Selector  InputPortWidth=4  IndexOptions=Index vector (dialog)  Indices=1  OutputSizes=1
  Switch1 : Switch  Criteria=u2 > Threshold
  q_mix_sign : Outport
  wires:
  qd/1 -> Quaternion Multiplication1/2
  Quaternion Multiplication1/1 -> Gain/1, Switch1/1, Selector1/1  "q_mix"
  Gain/1 -> Switch1/3
  Selector1/1 -> GreaterThan2/1
  GreaterThan2/1 -> Switch1/2
  Constant1/1 -> GreaterThan2/2
  Quaternion Inverse/1 -> Quaternion Multiplication1/1
  qd_red_update/1 -> Quaternion Inverse/1
  Switch1/1 -> q_mix_sign/1  "q_mix_sign"

== system test_bu01_2018b/角度控制器/求取航向衰减后的期望四元数/获取地球系下当前机体系Z轴矢量 ==
  ang : Inport
  Quaternion Normalize1 : sharedutil/Quaternion Normalize  aMode=aMode
      settings: SourceProductName=Aerospace Blockset  SourceProductBaseCode=AE
  Quaternions to Direction Cosine Matrix1 : sharedtransform/Quaternions to  Direction Cosine Matrix  aMode=aMode
      settings: SourceProductName=Aerospace Blockset  SourceProductBaseCode=AE
  Rotation Angles to Quaternions : sharedtransform/Rotation Angles to Quaternions  rotationOrder=XYZ  aMode=aMode
      settings: SourceProductName=Aerospace Blockset  SourceProductBaseCode=AE
  提取机体系Z轴在 导航系下的矢量1 : Selector  NumberOfDimensions=2  InputPortWidth=3  IndexOptions=Index vector (dialog),Index vector (dialog)  Indices=3,[1 2 3]  OutputSizes=1,1
  q : Outport
  e_z : Outport  Port=2
  wires:
  Quaternions to Direction Cosine Matrix1/1 -> 提取机体系Z轴在 导航系下的矢量1/1
  Quaternion Normalize1/1 -> q/1, Quaternions to Direction Cosine Matrix1/1
  Rotation Angles to Quaternions/1 -> Quaternion Normalize1/1
  ang/1 -> Rotation Angles to Quaternions/1
  提取机体系Z轴在 导航系下的矢量1/1 -> e_z/1

== system test_bu01_2018b/角度控制器/求取航向衰减后的期望四元数/获取地球系下期望机体系Z轴矢量 ==
  exp : Inport
  Quaternion Normalize : sharedutil/Quaternion Normalize  aMode=aMode
      settings: SourceProductName=Aerospace Blockset  SourceProductBaseCode=AE
  Quaternions to Direction Cosine Matrix : sharedtransform/Quaternions to  Direction Cosine Matrix  aMode=aMode
      settings: SourceProductName=Aerospace Blockset  SourceProductBaseCode=AE
  Rotation Angles to Quaternions1 : sharedtransform/Rotation Angles to Quaternions  rotationOrder=XYZ  aMode=aMode
      settings: SourceProductName=Aerospace Blockset  SourceProductBaseCode=AE
  提取机体系Z轴在 导航系下的矢量 : Selector  NumberOfDimensions=2  InputPortWidth=3  IndexOptions=Index vector (dialog),Index vector (dialog)  Indices=3,[1 2 3]  OutputSizes=1,1
  e_z_d : Outport
  "qd " : Outport  Port=2
  wires:
  Rotation Angles to Quaternions1/1 -> Quaternion Normalize/1
  Quaternion Normalize/1 -> "qd "/1, Quaternions to Direction Cosine Matrix/1
  Quaternions to Direction Cosine Matrix/1 -> 提取机体系Z轴在 导航系下的矢量/1
  提取机体系Z轴在 导航系下的矢量/1 -> e_z_d/1
  exp/1 -> Rotation Angles to Quaternions1/1

== system test_bu01_2018b/角度控制器/求取航向衰减后的期望四元数/计算航向衰减后的期望四元数 ==
  yaw_w : Inport
  q_red_update : Inport  Port=2
  q_mix_sign : Inport  Port=3
  Acos : Trigonometry  Operator=acos
  Acos1 : Trigonometry  Operator=asin
  Constant3 : Constant  Value=0
  Cos : Trigonometry  Operator=cos
  Cos1 : Trigonometry
  Demux1 : Demux  Outputs=2
  Mux : Mux
  Product : Product
  Product1 : Product
  Quaternion Multiplication2 : aerolibutil/Quaternion Multiplication
  Saturation : Saturate  UpperLimit=1  LowerLimit=-1
  Selector2 : Selector  InputPortWidth=4  IndexOptions=Index vector (dialog)  Indices=[1 4]  OutputSizes=1
  qd : Outport
  wires:
  Product/1 -> Cos/1
  Cos/1 -> Mux/1
  Cos1/1 -> Mux/4
  Saturation/1 -> Demux1/1
  yaw_w/1 -> Product1/2, Product/1
  Acos/1 -> Product/2
  Demux1/1 -> Acos/1
  Product1/1 -> Cos1/1
  Mux/1 -> Quaternion Multiplication2/2
  Quaternion Multiplication2/1 -> qd/1  "qd"
  Constant3/1 -> Mux/3, Mux/2
  Acos1/1 -> Product1/1
  q_red_update/1 -> Quaternion Multiplication2/1
  Demux1/2 -> Acos1/1
  Selector2/1 -> Saturation/1
  q_mix_sign/1 -> Selector2/1

== system test_bu01_2018b/bu01_model/动力系统模型/Motor1_TM_P/TM1654P  ==
  Vb : Inport  PortDimensions=3
  Wb : Inport  Port=2  PortDimensions=3
  Ax : Inport  Port=3  PortDimensions=3
  Density : Inport  Port=4  PortDimensions=1
  Ns : Inport  Port=5  PortDimensions=1
  Bus Selector : BusSelector  OutputSignals=FM,Tq,Izz
  Bus Selector1 : BusSelector  OutputSignals=Fb,Mb
  Bus Creator : BusCreator  Inputs=5
  螺旋桨模型 : Subsystem  mask{Izz=0.00024, D=0.406, Fratio=1.125, Mratio=0.975}
      mask prompts: Izz "螺旋桨惯量Izz"; D "螺旋桨直径D"; Fratio "推力系数Fratio"; Mratio "力矩系数Mratio"
      mask Display: disp('螺旋桨模型')
  Fb : Outport
  Mb : Outport  Port=2
  Tq : Outport  Port=3
  Izz : Outport  Port=4
  wires:
  Bus Selector/1 -> Bus Selector1/1  "<FM>"
  Bus Selector/3 -> Izz/1  "<Izz>"
  Bus Selector1/2 -> Mb/1  "<Mb>"
  Wb/1 -> Bus Creator/2  "Wb"
  Bus Selector1/1 -> Fb/1  "<Fb>"
  Ax/1 -> Bus Creator/3  "Ax"
  Density/1 -> Bus Creator/4  "Density"
  Bus Selector/2 -> Tq/1  "<Tq>"
  螺旋桨模型/1(TM_OUT) -> Bus Selector/1
  Vb/1 -> Bus Creator/1  "Vb"
  Ns/1 -> Bus Creator/5  "Ns"
  Bus Creator/1 -> 螺旋桨模型/1(In1)

== system test_bu01_2018b/bu01_model/动力系统模型/Motor1_TM_P/TMU5KV400  ==
  Um : Inport  PortDimensions=1
  Tq : Inport  Port=2  PortDimensions=1
  Izz : Inport  Port=3  PortDimensions=1
  Bus Selector : BusSelector  OutputSignals=Im,RPM
  Bus Creator : BusCreator  Inputs=3
  DCMotor : Subsystem  mask{L=0.0053, Km=0.024, Kemf=0.024, Imzz=0.00002, Ra=0.113, I0=0.725}
      mask prompts: L "电感值L"; Km "转矩常量Km"; Kemf "反电动势Kemf"; Imzz "转子惯量Imzz"; Ra "电动机内阻Ra"; I0 "空载电流I0"
      mask Display: disp('DCMotor')
  Im : Outport
  RPM : Outport  Port=2
  wires:
  Bus Selector/2 -> RPM/1  "<RPM>"
  Bus Selector/1 -> Im/1  "<Im>"
  DCMotor/1(Out1) -> Bus Selector/1
  Um/1 -> Bus Creator/1  "Um"
  Bus Creator/1 -> DCMotor/1(In1)
  Izz/1 -> Bus Creator/3  "Izz"
  Tq/1 -> Bus Creator/2  "Tq"

== system test_bu01_2018b/bu01_model/动力系统模型/Motor2_TM_N/TM1654N  ==
  Vb : Inport  PortDimensions=3
  Wb : Inport  Port=2  PortDimensions=3
  Ax : Inport  Port=3  PortDimensions=3
  Density : Inport  Port=4  PortDimensions=1
  Ns : Inport  Port=5  PortDimensions=1
  Bus Selector : BusSelector  OutputSignals=FM,Tq,Izz
  Bus Selector1 : BusSelector  OutputSignals=Fb,Mb
  Bus Creator : BusCreator  Inputs=5
  螺旋桨模型 : Subsystem  mask{Izz=0.00024, D=0.406, Fratio=1.125, Mratio=0.975}
      mask prompts: Izz "螺旋桨惯量Izz"; D "螺旋桨直径D"; Fratio "推力系数Fratio"; Mratio "力矩系数Mratio"
      mask Display: disp('螺旋桨模型')
  Fb : Outport
  Mb : Outport  Port=2
  Tq : Outport  Port=3
  Izz : Outport  Port=4
  wires:
  Bus Selector/2 -> Tq/1  "<Tq>"
  Bus Selector1/1 -> Fb/1  "<Fb>"
  Bus Selector/1 -> Bus Selector1/1  "<FM>"
  Bus Selector/3 -> Izz/1  "<Izz>"
  Bus Selector1/2 -> Mb/1  "<Mb>"
  螺旋桨模型/1(TM_OUT) -> Bus Selector/1
  Vb/1 -> Bus Creator/1  "Vb"
  Bus Creator/1 -> 螺旋桨模型/1(In1)
  Wb/1 -> Bus Creator/2  "Wb"
  Ns/1 -> Bus Creator/5  "Ns"
  Ax/1 -> Bus Creator/3  "Ax"
  Density/1 -> Bus Creator/4  "Density"

== system test_bu01_2018b/bu01_model/动力系统模型/Motor2_TM_N/TMU5KV400  ==
  Um : Inport  PortDimensions=1
  Tq : Inport  Port=2  PortDimensions=1
  Izz : Inport  Port=3  PortDimensions=1
  Bus Selector : BusSelector  OutputSignals=Im,RPM
  Bus Creator : BusCreator  Inputs=3
  DCMotor : Subsystem  mask{L=0.0053, Km=0.024, Kemf=0.024, Imzz=0.00002, Ra=0.113, I0=0.725}
      mask prompts: L "电感值L"; Km "转矩常量Km"; Kemf "反电动势Kemf"; Imzz "转子惯量Imzz"; Ra "电动机内阻Ra"; I0 "空载电流I0"
      mask Display: disp('DCMotor')
  Im : Outport
  RPM : Outport  Port=2
  wires:
  Bus Selector/2 -> RPM/1  "<RPM>"
  Bus Selector/1 -> Im/1  "<Im>"
  DCMotor/1(Out1) -> Bus Selector/1
  Um/1 -> Bus Creator/1  "Um"
  Bus Creator/1 -> DCMotor/1(In1)
  Izz/1 -> Bus Creator/3  "Izz"
  Tq/1 -> Bus Creator/2  "Tq"

== system test_bu01_2018b/bu01_model/动力系统模型/Motor3_TM_P/TM1654P  ==
  Vb : Inport  PortDimensions=3
  Wb : Inport  Port=2  PortDimensions=3
  Ax : Inport  Port=3  PortDimensions=3
  Density : Inport  Port=4  PortDimensions=1
  Ns : Inport  Port=5  PortDimensions=1
  Bus Selector : BusSelector  OutputSignals=FM,Tq,Izz
  Bus Selector1 : BusSelector  OutputSignals=Fb,Mb
  Bus Creator : BusCreator  Inputs=5
  螺旋桨模型 : Subsystem  mask{Izz=0.00024, D=0.406, Fratio=1.125, Mratio=0.975}
      mask prompts: Izz "螺旋桨惯量Izz"; D "螺旋桨直径D"; Fratio "推力系数Fratio"; Mratio "力矩系数Mratio"
      mask Display: disp('螺旋桨模型')
  Fb : Outport
  Mb : Outport  Port=2
  Tq : Outport  Port=3
  Izz : Outport  Port=4
  wires:
  Bus Selector/1 -> Bus Selector1/1  "<FM>"
  Bus Selector/3 -> Izz/1  "<Izz>"
  Bus Selector1/2 -> Mb/1  "<Mb>"
  Wb/1 -> Bus Creator/2  "Wb"
  Bus Selector1/1 -> Fb/1  "<Fb>"
  Ax/1 -> Bus Creator/3  "Ax"
  Density/1 -> Bus Creator/4  "Density"
  Bus Selector/2 -> Tq/1  "<Tq>"
  螺旋桨模型/1(TM_OUT) -> Bus Selector/1
  Vb/1 -> Bus Creator/1  "Vb"
  Ns/1 -> Bus Creator/5  "Ns"
  Bus Creator/1 -> 螺旋桨模型/1(In1)

== system test_bu01_2018b/bu01_model/动力系统模型/Motor3_TM_P/TMU5KV400  ==
  Um : Inport  PortDimensions=1
  Tq : Inport  Port=2  PortDimensions=1
  Izz : Inport  Port=3  PortDimensions=1
  Bus Selector : BusSelector  OutputSignals=Im,RPM
  Bus Creator : BusCreator  Inputs=3
  DCMotor : Subsystem  mask{L=0.0053, Km=0.024, Kemf=0.024, Imzz=0.00002, Ra=0.113, I0=0.725}
      mask prompts: L "电感值L"; Km "转矩常量Km"; Kemf "反电动势Kemf"; Imzz "转子惯量Imzz"; Ra "电动机内阻Ra"; I0 "空载电流I0"
      mask Display: disp('DCMotor')
  Im : Outport
  RPM : Outport  Port=2
  wires:
  Bus Selector/2 -> RPM/1  "<RPM>"
  Bus Selector/1 -> Im/1  "<Im>"
  DCMotor/1(Out1) -> Bus Selector/1
  Um/1 -> Bus Creator/1  "Um"
  Bus Creator/1 -> DCMotor/1(In1)
  Izz/1 -> Bus Creator/3  "Izz"
  Tq/1 -> Bus Creator/2  "Tq"

== system test_bu01_2018b/bu01_model/动力系统模型/Motor4_TM_N/TM1654N  ==
  Vb : Inport  PortDimensions=3
  Wb : Inport  Port=2  PortDimensions=3
  Ax : Inport  Port=3  PortDimensions=3
  Density : Inport  Port=4  PortDimensions=1
  Ns : Inport  Port=5  PortDimensions=1
  Bus Selector : BusSelector  OutputSignals=FM,Tq,Izz
  Bus Selector1 : BusSelector  OutputSignals=Fb,Mb
  Bus Creator : BusCreator  Inputs=5
  螺旋桨模型 : Subsystem  mask{Izz=0.00024, D=0.406, Fratio=1.125, Mratio=0.975}
      mask prompts: Izz "螺旋桨惯量Izz"; D "螺旋桨直径D"; Fratio "推力系数Fratio"; Mratio "力矩系数Mratio"
      mask Display: disp('螺旋桨模型')
  Fb : Outport
  Mb : Outport  Port=2
  Tq : Outport  Port=3
  Izz : Outport  Port=4
  wires:
  Bus Selector/2 -> Tq/1  "<Tq>"
  Bus Selector1/1 -> Fb/1  "<Fb>"
  Bus Selector/1 -> Bus Selector1/1  "<FM>"
  Bus Selector/3 -> Izz/1  "<Izz>"
  Bus Selector1/2 -> Mb/1  "<Mb>"
  螺旋桨模型/1(TM_OUT) -> Bus Selector/1
  Vb/1 -> Bus Creator/1  "Vb"
  Bus Creator/1 -> 螺旋桨模型/1(In1)
  Wb/1 -> Bus Creator/2  "Wb"
  Ns/1 -> Bus Creator/5  "Ns"
  Ax/1 -> Bus Creator/3  "Ax"
  Density/1 -> Bus Creator/4  "Density"
